simulink model "open_loop_linear_ss"  (R2018b)
settings: Solver=FixedStepAuto  StartTime=0.0  StopTime=10.0  FixedStep=1/100  RelTol=1e-3  AbsTol=1e-3
model workspace: external: MATLAB File params.m (data not in the file)
values from neighbouring files (symbols this model uses):
  b = 1e-9    (= 1e-09)    [linear_manual.m]
  g = 9.81    [linear_manual.m]
  m = 0.027    [linear_manual.m]
libraries: nesl_utility x7
settings Model: Creator=Jocke  LastModifiedBy=BARIS
settings SolverCC: AutoScaleAbsTol=off
settings SFSimCC: SimUseLocalCustomCode=off
settings RTWCC: RTWUseLocalCustomCode=off
settings CodeAppCC: StateflowObjectComments=on
settings SimscapeCC: SimscapeNormalizeSystem=off  SimscapeLogType=all  SimscapeLogDataHistory=10000

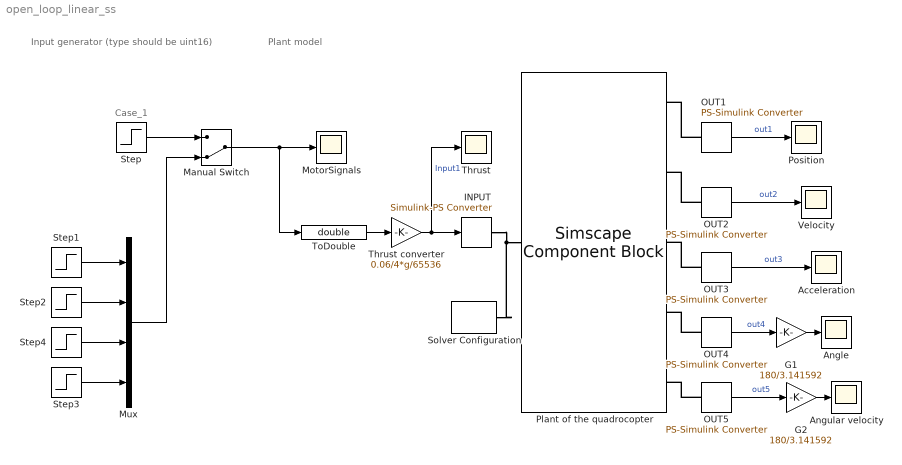
== system open_loop_linear_ss ==
  note: Case_1
  note: Input generator
      | (type should be uint16)
  note: Plant model
  Acceleration : Scope
  Angle : Scope
  Angular velocity : Scope
  G1 : Gain  Gain=180/3.141592
  G2 : Gain  Gain=180/3.141592
  INPUT : nesl_utility/Simulink-PS Converter  PhysicalDomain=network_engine_domain  SubClassName=ps_input  LeftPortType=input  RightPortType=output  PseudoPeriodic=off  Frequencies=[]  NoiseDistribution=none  NoiseParameters=[]  Unit=1  AffineConversion=off  FilteringAndDerivatives=zero  SimscapeFilterOrder=1  InputFilterTimeConstant=0.001  UdotUserProvided=1
  Manual Switch : ManualSwitch  CurrentSetting=0
  MotorSignals : Scope
  Mux : Mux
  OUT{1..5} (5 alike) : nesl_utility/PS-Simulink Converter  PhysicalDomain=network_engine_domain  SubClassName=ps_output  LeftPortType=input  RightPortType=output  PseudoPeriodic=off  Frequencies=[]  Unit=1  AffineConversion=off
  Plant of the quadrocopter : SimscapeComponentBlock  SourceFile=plant  ComponentPath=plant  ComponentVariants=plant  ComponentVariantNames=plant  ClassName=plant  SchemaVersion=1  m=m kg  g=g m/s^2  d=d m  b=b  k=1e-9 m
      settings: CopyFcn=simscape.engine.sli.internal.componentblockcallback(gcbh,'COPY')  PreCopyFcn=simscape.engine.sli.internal.componentblockcallback(gcbh,'PRECOPY')  PreDeleteFcn=simscape.engine.sli.internal.componentblockcallback(gcbh,'PREDELETE')
      mask Type: Plant of quadrocopter
  Position : Scope
  Solver Configuration : nesl_utility/Solver Configuration  PhysicalDomain=network_engine_domain  SubClassName=solver  LeftPortType=input  RightPortType=generic  Tones=[]  Harmonics=[]  SimulateNoise=off  Profile=off  UseLocalSampling=off  EnableSwitchedLinearOptims=on  FrequencyDomain=off  UseCCode=off  RelTol=0.001  AbsTol=1e-06  MinStep=1e-09  ToWorkspace=off  RevertToSquareIcSolve=off  NumHomotopyIterations=100  PhasorMode=off  PhasorModeNumHarmonics=1  DoDC=off  ResidualTolerance=1e-09  UseLocalSolver=off  LocalSolverChoice=NE_BACKWARD_EULER_ADVANCER  LocalSolverSampleTime=0.001  DoFixedCost=off  MaxNonlinIter=3  MaxModeIter=2  LinearAlgebra=Sparse  EquationFormulation=NE_TIME_EF  DelaysMemoryBudget=1024  AutomaticFiltering=on  FilteringTimeConstant=0.001  PartitionStorageMethod=AS_NEEDED  PartitionMemoryBudget=1024
  Step : Step  Time=4  Before=[0;0;0;0]  After=[10;10;0;0]  SampleTime=0
  Step1 : Step  Time=4  After=1000  SampleTime=0
  Step2 : Step  Time=0  After=0  SampleTime=0
  Step3 : Step  Time=0  After=0  SampleTime=0
  Step4 : Step  Time=6  After=2000  SampleTime=0
  Thrust : Scope
  Thrust converter : Gain  Gain=0.06/4*g/65536
  ToDouble : DataTypeConversion  OutDataTypeStr=double  RndMeth=Round  SaturateOnIntegerOverflow=on
  Velocity : Scope
  wires:
  G1/1 -> Angle/1
  G2/1 -> Angular velocity/1
  ToDouble/1 -> Thrust converter/1
  Thrust converter/1 -> Thrust/1, INPUT/1  "Input1"
  OUT1/1 -> Position/1  "out1"
  OUT5/1 -> G2/1  "out5"
  OUT4/1 -> G1/1  "out4"
  OUT3/1 -> Acceleration/1  "out3"
  OUT2/1 -> Velocity/1  "out2"
  Step/1 -> Manual Switch/1
  Manual Switch/1 -> ToDouble/1, MotorSignals/1
  Mux/1 -> Manual Switch/2
  Step1/1 -> Mux/1
  Step2/1 -> Mux/2
  Step4/1 -> Mux/3
  Step3/1 -> Mux/4
  connections:
  Plant of the quadrocopter/LConn1 -- INPUT/RConn1 -- Solver Configuration/RConn1
  OUT1/LConn1 -- Plant of the quadrocopter/RConn1
  OUT2/LConn1 -- Plant of the quadrocopter/RConn2
  OUT3/LConn1 -- Plant of the quadrocopter/RConn3
  OUT4/LConn1 -- Plant of the quadrocopter/RConn4
  OUT5/LConn1 -- Plant of the quadrocopter/RConn5
